simulink model "Motor_Model"  (Simulink 8.8)
settings: Solver=ode45  StartTime=0.0  StopTime=10.0  RelTol=1e-3  EnableMultiTasking=on
undefined symbols (not defined in the file or in its folder): b, J, K, L, R
settings Model: SuppressorTable=22 serialization::archive 11 0 3 0 0 0 11 0  Creator=maen  LastModifiedBy=aniket
settings OptimizationCC: ExpressionDepthLimit=2147483647

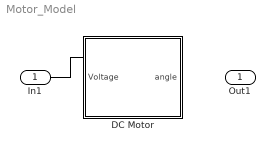
== system Motor_Model ==
  In1 : Inport
  DC Motor : Subsystem
  Out1 : Outport
  wires:
  In1/1 -> ?
  ? -> Out1/1

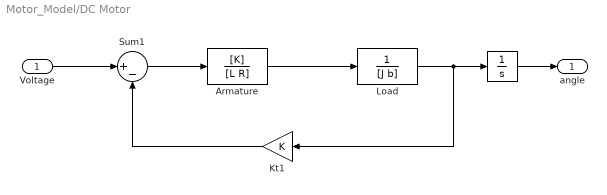
== system Motor_Model/DC Motor ==
  "Voltage " : Inport
  " " : Integrator
  Armature : TransferFcn  Numerator=[K]  Denominator=[L R]
  Kt1 : Gain  Gain=K
  Load : TransferFcn  Denominator=[J b]
  Sum1 : Sum  Inputs=|+-
  " angle" : Outport
  wires:
  Armature/1 -> Load/1
  Load/1 -> Kt1/1, " "/1
  "Voltage "/1 -> Sum1/1
  Sum1/1 -> Armature/1
  Kt1/1 -> Sum1/2
  " "/1 -> " angle"/1
